simulink model "testmodel1_org"  (Simulink 10.0)
settings: Solver=ode3  StartTime=0.0  StopTime=10.0  RelTol=1e-3  EnableMultiTasking=on
settings Model: Creator=Bryan  LastModifiedBy=annonymous
settings DataIOCC: LimitDataPoints=on
settings DebuggingCC: UnderspecifiedInitializationDetection=Simplified  MergeDetectMultiDrivingBlocksExec=error  SolverPrmCheckMsg=warning
settings RTWCC: Description=Create Visual C/C++ Solution File for Simulink Coder  TemplateMakefile=RTW.MSVCBuild  GenerateReport=on  LaunchReport=on
settings CodeAppCC: ForceParamTrailComments=on  MATLABSourceComments=on
settings GRTTargetCC: GeneratePreprocessorConditionals=Disable all  CombineOutputUpdateFcns=on  MatFileLogging=off  GRTInterface=off
settings ConfigComp: CovExternalEMLEnable=off  CovSFcnEnable=off

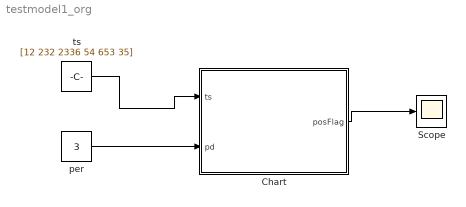
== system testmodel1_org ==
  Chart : Stateflow chart  TreatAsAtomicUnit=on
  Scope : Scope
  "per  " : Constant  Value=3
  ts : Constant  Value=[12 232 2336 54 653 35]  VectorParams1D=off
  wires:
  Chart/1(posFlag) -> Scope/1
  ts/1 -> Chart/1(ts)
  "per  "/1 -> Chart/2(pd)

== stateflow chart Chart ==
  state buy
    en: posFlag=1
  state sell
    en: posFlag=-1
  (default) -> (junction 13) : {avg=testMovAvg(ts,pd)}
  sell -> (junction 13)
  (junction 13) -> sell [order 2] : [avg>50]
  buy -> (junction 13)
  (junction 13) -> buy [order 1] : [avg<50]
  data: x function_input double; ped function_input double =ped; avgNum function_output double; posFlag output double size=1; ts input double; pd input double; avg local double
  function avgNum=testMovAvg(x,ped):
    | function avgNum=testMovAvg(x,ped)
    | %ensure out variable does not cofnflict with other model objects 
    | %this directive is need to add input and output on Stateflow chart block!
    | %#codegen
    | avgNum = 0; %must define for code generation
    | avgNum = sum(x)/ped;
